simulink model "Demo_CarRealTime2D_cs"  (R2014b)
settings: Solver=ode5  SolverMode=SingleTasking  StartTime=0.0  StopTime=inf  FixedStep=1/1000  RelTol=1e-3
PreLoadFcn:
  | mbxruntime.callbacks.PreLoadFcn(bdroot);
  | check_NUTS_defined;
  | assignin('base',['model_closed_' bdroot],false);
  | addpath('../includes_AEBS');
PostLoadFcn:
  | mbxruntime.callbacks.PostLoadFcn(bdroot);
InitFcn:
  | mbxruntime.callbacks.InitFcn(bdroot);
StartFcn:
  | mbxruntime.callbacks.StartFcn(bdroot);
StopFcn:
  | mbxruntime.callbacks.StopFcn(bdroot);;
  | 
model workspace: external: MAT-File .\Demo_CarRealTime2D_cs_hws.mat (data not in the file)
undefined symbols (not defined in the file or in its folder): Driver_Demands, mbxruntime, tabledata, vicrt_initcallback, vicrt_initmexcallback, vicrt_simulationmanager, warningInitialVelocity, x0
undefined symbols (not defined in the file): Demo_CarRealTime2D_cs_007c1c37f387f47f, Demo_CarRealTime2D_cs_085a64a83ba38cec, Demo_CarRealTime2D_cs_0a7f542d3fc7ab9f, Demo_CarRealTime2D_cs_0d7c72cfaa56dff7, Demo_CarRealTime2D_cs_0de07b35068e3828, Demo_CarRealTime2D_cs_17f4d381375cce95, Demo_CarRealTime2D_cs_1db40a09b08215a9, Demo_CarRealTime2D_cs_2bfa3850c176687b, Demo_CarRealTime2D_cs_35a34f1ba6ce4a22, Demo_CarRealTime2D_cs_378cc77e08d643fb, Demo_CarRealTime2D_cs_409b5c3befba0000, Demo_CarRealTime2D_cs_42628ca5bb62d2f3, Demo_CarRealTime2D_cs_56554a2db408a7f8, Demo_CarRealTime2D_cs_59527455249d7429, Demo_CarRealTime2D_cs_5983ee1b8112afac, Demo_CarRealTime2D_cs_5b5ebcf3ed7bf8e6, Demo_CarRealTime2D_cs_63cbe7fbe16cd5d9, Demo_CarRealTime2D_cs_6e17b9adbf989abf, Demo_CarRealTime2D_cs_6f662a34e5d9a196, Demo_CarRealTime2D_cs_75c4ee8892821e19, Demo_CarRealTime2D_cs_7c64486355814be2, Demo_CarRealTime2D_cs_849809550a2230ef, Demo_CarRealTime2D_cs_87f899bcbe16d8f5, Demo_CarRealTime2D_cs_8e7b50dac25b68a2, Demo_CarRealTime2D_cs_94938e5260f139b3, Demo_CarRealTime2D_cs_983acc940698d1d1, Demo_CarRealTime2D_cs_9d554c72797f76fd, Demo_CarRealTime2D_cs_9d747ee2f15c057f, Demo_CarRealTime2D_cs_ad62a2084d31e898, Demo_CarRealTime2D_cs_b56c8c5f000d30f0, Demo_CarRealTime2D_cs_b95f1b7356e926cc, Demo_CarRealTime2D_cs_BMW_X5_1_Path_pathUniqueID, Demo_CarRealTime2D_cs_BMW_Z3_2_Dynamics_Empty_STATE_BMW_Z3_2_x0, Demo_CarRealTime2D_cs_BMW_Z3_2_Dynamics_Empty_STATE_BMW_Z3_2_y0, Demo_CarRealTime2D_cs_BMW_Z3_2_Dynamics_Empty_STATE_BMW_Z3_2_z0, Demo_CarRealTime2D_cs_BMW_Z3_Path_pathUniqueID, Demo_CarRealTime2D_cs_BMW_Z3_SpeedProfile_speedProfileUniqueID, Demo_CarRealTime2D_cs_c8847ab2e5633224, Demo_CarRealTime2D_cs_c9a0d701286b93fb, Demo_CarRealTime2D_cs_ce758cae7dd1b283, Demo_CarRealTime2D_cs_CrossingPedestrian_Path_pathUniqueID, Demo_CarRealTime2D_cs_CuttingInVehicle_Path_pathUniqueID, Demo_CarRealTime2D_cs_d901ab1c1d2e40bc, Demo_CarRealTime2D_cs_dff70430e5a00a86, Demo_CarRealTime2D_cs_ef038a4f619ad32e, Demo_CarRealTime2D_cs_Female_OverweightAni_1_Path_pathUniqueID, Demo_CarRealTime2D_cs_Ford_Fiesta_1_Path_pathUniqueID, Demo_CarRealTime2D_cs_Ford_FocusWagon_Path_pathUniqueID, Demo_CarRealTime2D_cs_Sphere_1_Dynamics_Empty_STATE_Sphere_1_x0, Demo_CarRealTime2D_cs_Sphere_1_Dynamics_Empty_STATE_Sphere_1_y0, Demo_CarRealTime2D_cs_Sphere_1_Dynamics_Empty_STATE_Sphere_1_z0, WheelL0, WheelL1, WheelR0, WheelR1
libraries: PreScanSimulinkLibrary x15, simulink x15, simulink_extras x15, PreScanUsefulBlocks x2, dspsigops x1
(part 17 of 17)

== system Demo_CarRealTime2D_cs/HostVehicle/Dynamics_UserSpecified/VI-CarRealTime/Input_Bus/Inputs/Mono_Element/Reboundstop_Spring ==
  BCReboundstop_Spring : BusCreator  Inputs=2
  front_def_val : Constant  Value=0
  rear_def_val : Constant  Value=0
  Reboundstop_Spring : Outport
  wires:
  rear_def_val/1 -> BCReboundstop_Spring/2  "rear"
  front_def_val/1 -> BCReboundstop_Spring/1  "front"
  BCReboundstop_Spring/1 -> Reboundstop_Spring/1  "Reboundstop_Spring"

== system Demo_CarRealTime2D_cs/HostVehicle/Dynamics_UserSpecified/VI-CarRealTime/Input_Bus/Inputs/Mono_Element/Reboundstop_Spring_activity_flag ==
  BCReboundstop_Spring_activity_flag : BusCreator  Inputs=2
  front_def_val : Constant
  rear_def_val : Constant
  Reboundstop_Spring_activity_flag : Outport
  wires:
  rear_def_val/1 -> BCReboundstop_Spring_activity_flag/2  "rear"
  front_def_val/1 -> BCReboundstop_Spring_activity_flag/1  "front"
  BCReboundstop_Spring_activity_flag/1 -> Reboundstop_Spring_activity_flag/1  "Reboundstop_Spring_activity_flag"

== system Demo_CarRealTime2D_cs/HostVehicle/Dynamics_UserSpecified/VI-CarRealTime/Input_Bus/Inputs/Mono_Element/Spring ==
  BCSpring : BusCreator  Inputs=2
  front_def_val : Constant  Value=0
  rear_def_val : Constant  Value=0
  Spring : Outport
  wires:
  rear_def_val/1 -> BCSpring/2  "rear"
  front_def_val/1 -> BCSpring/1  "front"
  BCSpring/1 -> Spring/1  "Spring"

== system Demo_CarRealTime2D_cs/HostVehicle/Dynamics_UserSpecified/VI-CarRealTime/Input_Bus/Inputs/Mono_Element/Spring_activity_flag ==
  BCSpring_activity_flag : BusCreator  Inputs=2
  front_def_val : Constant
  rear_def_val : Constant
  Spring_activity_flag : Outport
  wires:
  rear_def_val/1 -> BCSpring_activity_flag/2  "rear"
  front_def_val/1 -> BCSpring_activity_flag/1  "front"
  BCSpring_activity_flag/1 -> Spring_activity_flag/1  "Spring_activity_flag"

== system Demo_CarRealTime2D_cs/HostVehicle/Dynamics_UserSpecified/VI-CarRealTime/Input_Bus/Inputs/Rear_Steering_Actuator_disp/str_swa ==
  BCstr_swa : BusCreator  Inputs=2
  left_def_val : Constant  Value=0
  right_def_val : Constant  Value=0
  str_swa : Outport
  wires:
  right_def_val/1 -> BCstr_swa/2  "right"
  left_def_val/1 -> BCstr_swa/1  "left"
  BCstr_swa/1 -> str_swa/1  "str_swa"

== system Demo_CarRealTime2D_cs/HostVehicle/Dynamics_UserSpecified/VI-CarRealTime/Input_Bus/Inputs/Steering/steer_at_spindle ==
  BCsteer_at_spindle : BusCreator
  L1_def_val : Constant  Value=0
  L2_def_val : Constant  Value=0
  R1_def_val : Constant  Value=0
  R2_def_val : Constant  Value=0
  steer_at_spindle : Outport
  wires:
  R2_def_val/1 -> BCsteer_at_spindle/4  "R2"
  R1_def_val/1 -> BCsteer_at_spindle/3  "R1"
  L2_def_val/1 -> BCsteer_at_spindle/2  "L2"
  L1_def_val/1 -> BCsteer_at_spindle/1  "L1"
  BCsteer_at_spindle/1 -> steer_at_spindle/1  "steer_at_spindle"

== system Demo_CarRealTime2D_cs/HostVehicle/Dynamics_UserSpecified/VI-CarRealTime/Input_Bus/Inputs/Subsystem_Activation/Internal_Brake_System_Activity ==
  BCInternal_Brake_System_Activity : BusCreator
  L1_def_val : Constant
  L2_def_val : Constant
  R1_def_val : Constant
  R2_def_val : Constant
  Internal_Brake_System_Activity : Outport
  wires:
  R2_def_val/1 -> BCInternal_Brake_System_Activity/4  "R2"
  R1_def_val/1 -> BCInternal_Brake_System_Activity/3  "R1"
  L2_def_val/1 -> BCInternal_Brake_System_Activity/2  "L2"
  L1_def_val/1 -> BCInternal_Brake_System_Activity/1  "L1"
  BCInternal_Brake_System_Activity/1 -> Internal_Brake_System_Activity/1  "Internal_Brake_System_Activity"

== system Demo_CarRealTime2D_cs/HostVehicle/Dynamics_UserSpecified/VI-CarRealTime/Input_Bus/Inputs/Subsystem_Activation/Tire_Force_x ==
  BCTire_Force_x : BusCreator
  L1_def_val : Constant
  L2_def_val : Constant
  R1_def_val : Constant
  R2_def_val : Constant
  Tire_Force_x : Outport
  wires:
  R2_def_val/1 -> BCTire_Force_x/4  "R2"
  R1_def_val/1 -> BCTire_Force_x/3  "R1"
  L2_def_val/1 -> BCTire_Force_x/2  "L2"
  L1_def_val/1 -> BCTire_Force_x/1  "L1"
  BCTire_Force_x/1 -> Tire_Force_x/1  "Tire_Force_x"

== system Demo_CarRealTime2D_cs/HostVehicle/Dynamics_UserSpecified/VI-CarRealTime/Input_Bus/Inputs/Subsystem_Activation/Tire_Force_y ==
  BCTire_Force_y : BusCreator
  L1_def_val : Constant
  L2_def_val : Constant
  R1_def_val : Constant
  R2_def_val : Constant
  Tire_Force_y : Outport
  wires:
  R2_def_val/1 -> BCTire_Force_y/4  "R2"
  R1_def_val/1 -> BCTire_Force_y/3  "R1"
  L2_def_val/1 -> BCTire_Force_y/2  "L2"
  L1_def_val/1 -> BCTire_Force_y/1  "L1"
  BCTire_Force_y/1 -> Tire_Force_y/1  "Tire_Force_y"

== system Demo_CarRealTime2D_cs/HostVehicle/Dynamics_UserSpecified/VI-CarRealTime/Input_Bus/Inputs/Subsystem_Activation/Tire_Force_z ==
  BCTire_Force_z : BusCreator
  L1_def_val : Constant
  L2_def_val : Constant
  R1_def_val : Constant
  R2_def_val : Constant
  Tire_Force_z : Outport
  wires:
  R2_def_val/1 -> BCTire_Force_z/4  "R2"
  R1_def_val/1 -> BCTire_Force_z/3  "R1"
  L2_def_val/1 -> BCTire_Force_z/2  "L2"
  L1_def_val/1 -> BCTire_Force_z/1  "L1"
  BCTire_Force_z/1 -> Tire_Force_z/1  "Tire_Force_z"

== system Demo_CarRealTime2D_cs/HostVehicle/Dynamics_UserSpecified/VI-CarRealTime/Input_Bus/Inputs/Subsystem_Activation/Tire_Moment_x ==
  BCTire_Moment_x : BusCreator
  L1_def_val : Constant
  L2_def_val : Constant
  R1_def_val : Constant
  R2_def_val : Constant
  Tire_Moment_x : Outport
  wires:
  R2_def_val/1 -> BCTire_Moment_x/4  "R2"
  R1_def_val/1 -> BCTire_Moment_x/3  "R1"
  L2_def_val/1 -> BCTire_Moment_x/2  "L2"
  L1_def_val/1 -> BCTire_Moment_x/1  "L1"
  BCTire_Moment_x/1 -> Tire_Moment_x/1  "Tire_Moment_x"

== system Demo_CarRealTime2D_cs/HostVehicle/Dynamics_UserSpecified/VI-CarRealTime/Input_Bus/Inputs/Subsystem_Activation/Tire_Moment_y ==
  BCTire_Moment_y : BusCreator
  L1_def_val : Constant
  L2_def_val : Constant
  R1_def_val : Constant
  R2_def_val : Constant
  Tire_Moment_y : Outport
  wires:
  R2_def_val/1 -> BCTire_Moment_y/4  "R2"
  R1_def_val/1 -> BCTire_Moment_y/3  "R1"
  L2_def_val/1 -> BCTire_Moment_y/2  "L2"
  L1_def_val/1 -> BCTire_Moment_y/1  "L1"
  BCTire_Moment_y/1 -> Tire_Moment_y/1  "Tire_Moment_y"

== system Demo_CarRealTime2D_cs/HostVehicle/Dynamics_UserSpecified/VI-CarRealTime/Input_Bus/Inputs/Subsystem_Activation/Tire_Moment_z ==
  BCTire_Moment_z : BusCreator
  L1_def_val : Constant
  L2_def_val : Constant
  R1_def_val : Constant
  R2_def_val : Constant
  Tire_Moment_z : Outport
  wires:
  R2_def_val/1 -> BCTire_Moment_z/4  "R2"
  R1_def_val/1 -> BCTire_Moment_z/3  "R1"
  L2_def_val/1 -> BCTire_Moment_z/2  "L2"
  L1_def_val/1 -> BCTire_Moment_z/1  "L1"
  BCTire_Moment_z/1 -> Tire_Moment_z/1  "Tire_Moment_z"

== system Demo_CarRealTime2D_cs/HostVehicle/Dynamics_UserSpecified/VI-CarRealTime/Input_Bus/Inputs/Third_Element/Damper_activity_flag ==
  BCDamper_activity_flag : BusCreator  Inputs=2
  front_def_val : Constant
  rear_def_val : Constant
  Damper_activity_flag : Outport
  wires:
  rear_def_val/1 -> BCDamper_activity_flag/2  "rear"
  front_def_val/1 -> BCDamper_activity_flag/1  "front"
  BCDamper_activity_flag/1 -> Damper_activity_flag/1  "Damper_activity_flag"

== system Demo_CarRealTime2D_cs/HostVehicle/Dynamics_UserSpecified/VI-CarRealTime/Input_Bus/Inputs/Third_Element/Damper_force ==
  BCDamper_force : BusCreator  Inputs=2
  front_def_val : Constant  Value=0
  rear_def_val : Constant  Value=0
  Damper_force : Outport
  wires:
  rear_def_val/1 -> BCDamper_force/2  "rear"
  front_def_val/1 -> BCDamper_force/1  "front"
  BCDamper_force/1 -> Damper_force/1  "Damper_force"

== system Demo_CarRealTime2D_cs/HostVehicle/Dynamics_UserSpecified/VI-CarRealTime/Input_Bus/Inputs/Third_Element/Spring ==
  BCSpring : BusCreator  Inputs=2
  front_def_val : Constant  Value=0
  rear_def_val : Constant  Value=0
  Spring : Outport
  wires:
  rear_def_val/1 -> BCSpring/2  "rear"
  front_def_val/1 -> BCSpring/1  "front"
  BCSpring/1 -> Spring/1  "Spring"

== system Demo_CarRealTime2D_cs/HostVehicle/Dynamics_UserSpecified/VI-CarRealTime/Input_Bus/Inputs/Third_Element/Spring_activity_flag ==
  BCSpring_activity_flag : BusCreator  Inputs=2
  front_def_val : Constant
  rear_def_val : Constant
  Spring_activity_flag : Outport
  wires:
  rear_def_val/1 -> BCSpring_activity_flag/2  "rear"
  front_def_val/1 -> BCSpring_activity_flag/1  "front"
  BCSpring_activity_flag/1 -> Spring_activity_flag/1  "Spring_activity_flag"

== system Demo_CarRealTime2D_cs/HostVehicle/Dynamics_UserSpecified/VI-CarRealTime/Input_Bus/Inputs/Tire_Force/Fx ==
  BCFx : BusCreator
  L1_def_val : Constant  Value=0
  L2_def_val : Constant  Value=0
  R1_def_val : Constant  Value=0
  R2_def_val : Constant  Value=0
  Fx : Outport
  wires:
  R2_def_val/1 -> BCFx/4  "R2"
  R1_def_val/1 -> BCFx/3  "R1"
  L2_def_val/1 -> BCFx/2  "L2"
  L1_def_val/1 -> BCFx/1  "L1"
  BCFx/1 -> Fx/1  "Fx"

== system Demo_CarRealTime2D_cs/HostVehicle/Dynamics_UserSpecified/VI-CarRealTime/Input_Bus/Inputs/Tire_Force/Fy ==
  BCFy : BusCreator
  L1_def_val : Constant  Value=0
  L2_def_val : Constant  Value=0
  R1_def_val : Constant  Value=0
  R2_def_val : Constant  Value=0
  Fy : Outport
  wires:
  R2_def_val/1 -> BCFy/4  "R2"
  R1_def_val/1 -> BCFy/3  "R1"
  L2_def_val/1 -> BCFy/2  "L2"
  L1_def_val/1 -> BCFy/1  "L1"
  BCFy/1 -> Fy/1  "Fy"

== system Demo_CarRealTime2D_cs/HostVehicle/Dynamics_UserSpecified/VI-CarRealTime/Input_Bus/Inputs/Tire_Force/Fz ==
  BCFz : BusCreator
  L1_def_val : Constant  Value=0
  L2_def_val : Constant  Value=0
  R1_def_val : Constant  Value=0
  R2_def_val : Constant  Value=0
  Fz : Outport
  wires:
  R2_def_val/1 -> BCFz/4  "R2"
  R1_def_val/1 -> BCFz/3  "R1"
  L2_def_val/1 -> BCFz/2  "L2"
  L1_def_val/1 -> BCFz/1  "L1"
  BCFz/1 -> Fz/1  "Fz"

== system Demo_CarRealTime2D_cs/HostVehicle/Dynamics_UserSpecified/VI-CarRealTime/Input_Bus/Inputs/Tire_Moment/Mx ==
  BCMx : BusCreator
  L1_def_val : Constant  Value=0
  L2_def_val : Constant  Value=0
  R1_def_val : Constant  Value=0
  R2_def_val : Constant  Value=0
  Mx : Outport
  wires:
  R2_def_val/1 -> BCMx/4  "R2"
  R1_def_val/1 -> BCMx/3  "R1"
  L2_def_val/1 -> BCMx/2  "L2"
  L1_def_val/1 -> BCMx/1  "L1"
  BCMx/1 -> Mx/1  "Mx"

== system Demo_CarRealTime2D_cs/HostVehicle/Dynamics_UserSpecified/VI-CarRealTime/Input_Bus/Inputs/Tire_Moment/My ==
  BCMy : BusCreator
  L1_def_val : Constant  Value=0
  L2_def_val : Constant  Value=0
  R1_def_val : Constant  Value=0
  R2_def_val : Constant  Value=0
  My : Outport
  wires:
  R2_def_val/1 -> BCMy/4  "R2"
  R1_def_val/1 -> BCMy/3  "R1"
  L2_def_val/1 -> BCMy/2  "L2"
  L1_def_val/1 -> BCMy/1  "L1"
  BCMy/1 -> My/1  "My"

== system Demo_CarRealTime2D_cs/HostVehicle/Dynamics_UserSpecified/VI-CarRealTime/Input_Bus/Inputs/Tire_Moment/Mz ==
  BCMz : BusCreator
  L1_def_val : Constant  Value=0
  L2_def_val : Constant  Value=0
  R1_def_val : Constant  Value=0
  R2_def_val : Constant  Value=0
  Mz : Outport
  wires:
  R2_def_val/1 -> BCMz/4  "R2"
  R1_def_val/1 -> BCMz/3  "R1"
  L2_def_val/1 -> BCMz/2  "L2"
  L1_def_val/1 -> BCMz/1  "L1"
  BCMz/1 -> Mz/1  "Mz"

== system Demo_CarRealTime2D_cs/HostVehicle/Dynamics_UserSpecified/VI-CarRealTime/Input_Bus/Inputs/Wheel_driving/moment ==
  BCmoment : BusCreator
  L1_def_val : Constant  Value=0
  L2_def_val : Constant  Value=0
  R1_def_val : Constant  Value=0
  R2_def_val : Constant  Value=0
  moment : Outport
  wires:
  R2_def_val/1 -> BCmoment/4  "R2"
  R1_def_val/1 -> BCmoment/3  "R1"
  L2_def_val/1 -> BCmoment/2  "L2"
  L1_def_val/1 -> BCmoment/1  "L1"
  BCmoment/1 -> moment/1  "moment"

== matlab function Demo_CarRealTime2D_cs/ToLegacyCollisionOutput/ToLegacyCollisionOutput ==
  data: in input; IDs output; Detections output
function [IDs, Detections]= ToLegacyCollisionOutput(in)
%#eml

MAX_OUTPUTS = 5;

IDs = zeros(MAX_OUTPUTS*2,1);
Detections = false(MAX_OUTPUTS, 1);

for i = 1 : min(length(in), MAX_OUTPUTS)
    if in(i).HEADER.valid == 1
        
         index = (i-1)*2 + 1;
         IDs(index)     = in(i).DATA.ObjectID1;
         IDs(index + 1) = in(i).DATA.ObjectID2;
         
         Detections(i) = true;
    end
end

== matlab function Demo_CarRealTime2D_cs/HostVehicle/PathFollower_Preview_1/LateralController/Calculate delta steering error/eml_delta_steering_error ==
  data: v_x_vehicle input; v_x_vehicle_Min input; t_Preview_LatCtrl input; delta_steeringwheeltotal output; v_y_vehicle input; yawrate_vehicle input; CorneringStiffness_Tyres_Front input; CorneringStiffness_Tyres_Rear input; m_vehicle_total input; inertia_z_vehicle_total input; e_Lat input size=10; Pos_x_CoG_Vehicle input; wheelbase input; RefreshCounter parameter
function delta_steeringwheeltotal = eml_delta_steering_error(v_x_vehicle,v_x_vehicle_Min,t_Preview_LatCtrl,v_y_vehicle,yawrate_vehicle,CorneringStiffness_Tyres_Front,CorneringStiffness_Tyres_Rear,m_vehicle_total,inertia_z_vehicle_total,e_Lat,Pos_x_CoG_Vehicle,wheelbase,RefreshCounter)

delta_steeringwheeltotal = emlfcn_delta_steering_error(v_x_vehicle,v_x_vehicle_Min,t_Preview_LatCtrl,v_y_vehicle,yawrate_vehicle,CorneringStiffness_Tyres_Front,CorneringStiffness_Tyres_Rear,m_vehicle_total,inertia_z_vehicle_total,e_Lat,Pos_x_CoG_Vehicle,wheelbase,RefreshCounter);

% end function

== matlab function Demo_CarRealTime2D_cs/HostVehicle/Vehicles Synchronization/Evaluate_Event_To_Trigger_CuttingVehicle/Actor_Filter [Only Triggers When the Desired Actor Comes Within The Sensor FOV] ==
  data: Range_IN input; Theta_IN input; ID_IN input; V_IN input; Heading_IN input; Actor_ID input; Range_OUT output; Theta_OUT output; ID_OUT output; V_OUT output; Heading_OUT output

%%%%%%%%%%%%%%%%%%%%%%%%%%%%%%%%%%%%%%%%%%%%%%%%%%%%%%%%%%%%%%%%%%%%%%%%%%%%%%%%%%%%%%%%%%%%%%%%%%%%%%%%%%%%%%%%%%%%%%%%%%%%%%%%  
%%%%%%%%%%%%%%%%%%%%%%%%%%%%%%%%%%%%%%%%%%%%%%%%%%%%%%%%%%%%%%%%%%%%%%%%%%%%%%%%%%%%%%%%%%%%%%%%%%%%%%%%%%%%%%%%%%%%%%%%%%%%%%%% 
 %  This function extracts specific object (pedestrian/no pedestrian) from all the detected objects (AIR sensor's outputs).    
 %  The inputs to this function are the AIR readings, as well as the constant value of Actor(Truck) ID to be defined by the user:                                              
%%%%%%%%%%%%%%%%%%%%%%%%%%%%%%%%%%%%%%%%%%%%%%%%%%%%%%%%%%%%%%%%%%%%%%%%%%%%%%%%%%%%%%%%%%%%%%%%%%%%%%%%%%%%%%%%%%%%%%%%%%%%%%%% 
%%%%%%%%%%%%%%%%%%%%%%%%%%%%%%%%%%%%%%%%%%%%%%%%%%%%%%%%%%%%%%%%%%%%%%%%%%%%%%%%%%%%%%%%%%%%%%%%%%%%%%%%%%%%%%%%%%%%%%%%%%%%%%%% 

function [Range_OUT,Theta_OUT,ID_OUT,V_OUT,Heading_OUT] = fcn(Range_IN,Theta_IN,ID_IN,V_IN,Heading_IN,Actor_ID)

% %% Variables Initialization%%

Range_OUT = 0;
Theta_OUT = 0;
ID_OUT = 0;
V_OUT = 0;
Heading_OUT = 0;

coder.extrinsic('disp')
coder.extrinsic('sprintf')

% Extraction %

%% Do not execute this script if Actor ID is set to 0 (inconsistent conditions).
%  Should this be the case, a warning message will be displayed in the Command Window and the scripts' outputs are set to 0 (No extraction will be performed)

if  Actor_ID == 0
    disp(sprintf('The objects selection criteria are not consistent.\nSet ''Actor ID'''))
    return
end

for i = 1:length(Range_IN)
    if ID_IN(i) == Actor_ID
        Range_OUT = Range_IN(i);
        Theta_OUT = Theta_IN(i);
        ID_OUT = ID_IN(i);
        V_OUT = V_IN(i);
        Heading_OUT = Heading_IN(i);
    end
end

== matlab function Demo_CarRealTime2D_cs/CuttingInVehicle/Trajectories1/Trajectory_Host_AllSystems/Embeded MATLAB S-Function/MATLAB Function ==
  data: gain input; offset input; y output; trajectory parameter; TimeStep parameter
% this function is provided for demo purposes. Before releasing this 
% code to customers, this code needs to be checked for correctness.

function y  = fcn(gain, offset, trajectory, TimeStep)
    %#codegen
 
    persistent local_time;
    persistent k; %compensation factor in time
    if isempty(local_time)
        local_time = 0;
        k=1;
    else
        local_time = local_time + 1/k*gain*TimeStep;
    end

    local_time = min(local_time, trajectory.final_time);
    v = interp1(trajectory.time, trajectory.data, local_time);
    if (local_time == trajectory.final_time)
        gain = 0;
    end
    
    persistent prev_pos;
    if isempty(prev_pos)
        prev_pos = v(1:3);      %x,y,z positions
    end
    
    persistent prev_offset;
    if isempty(prev_offset)
        prev_offset = offset;
    end 
    
    %correction angle for offset changes
    distance = norm(v(1:3)-prev_pos);
    beta = 0;
    if distance > 0.0
        z = min(max((offset-prev_offset)/distance, -1),1);
        beta = atan(z);
    end
    
    delta_alpha_traj = prev_pos(3)-v(3);
    delta_dist = norm(v(1:3) - prev_pos(1:3));
    if (delta_alpha_traj)
        k = offset / (delta_dist / delta_alpha_traj) + 1;
    else
        k = 1;
    end
    
    prev_pos = v(1:3);
    prev_offset = offset;

    xo = -offset*sin(v(6));
    yo = offset*cos(v(6));
    y = [v(1:6)+[xo yo 0 0 0 beta], v(7:18)*gain]';
%endfunction
